simulink model "BasicFF"  (R2016a)
settings: Solver=FixedStepAuto  StartTime=0.0  StopTime=48*60  FixedStep=1  RelTol=1e-3
values from neighbouring files (symbols this model uses):
  Ki = -0.075*(1+Ki_uncertainty)    (= -0.075)    [DiabetesVariables.m]
  Ki0 = -0.075    [Qdesign.m]
  Km = 4    [DiabetesVariables.m]
  Tdi = 25    [DiabetesVariables.m]
  Tdm = 15    [DiabetesVariables.m]
  Ti = 140    [DiabetesVariables.m]
  Tm = 50    [DiabetesVariables.m]
settings Model: Creator=benma  LastModifiedBy=benma

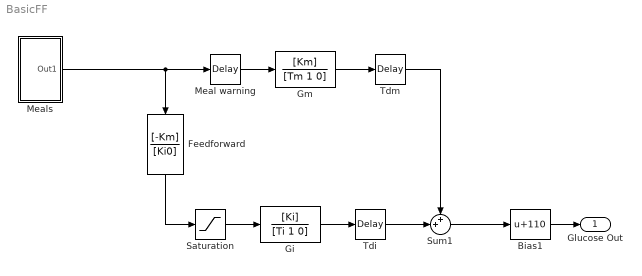
== system BasicFF ==
  Bias1 : Bias  Bias=110
  Feedforward : TransferFcn  Numerator=[-Km]  Denominator=[Ki0]
  Gi : TransferFcn  Numerator=[Ki]  Denominator=[Ti 1 0]
  Gm : TransferFcn  Numerator=[Km]  Denominator=[Tm 1 0]
  Meal warning : TransportDelay  DelayTime=10
  Meals : Subsystem
  Saturation : Saturate  UpperLimit=166  LowerLimit=0
  Sum1 : Sum  Inputs=++|
  Tdi : TransportDelay  DelayTime=Tdi
  Tdm : TransportDelay  DelayTime=Tdm
  Glucose Out : Outport
  wires:
  Gi/1 -> Tdi/1
  Tdi/1 -> Sum1/2
  Gm/1 -> Tdm/1
  Sum1/1 -> Bias1/1
  Tdm/1 -> Sum1/1
  Bias1/1 -> Glucose Out/1
  Saturation/1 -> Gi/1
  Feedforward/1 -> Saturation/1
  Meals/1(Out1) -> Meal warning/1, Feedforward/1
  Meal warning/1 -> Gm/1

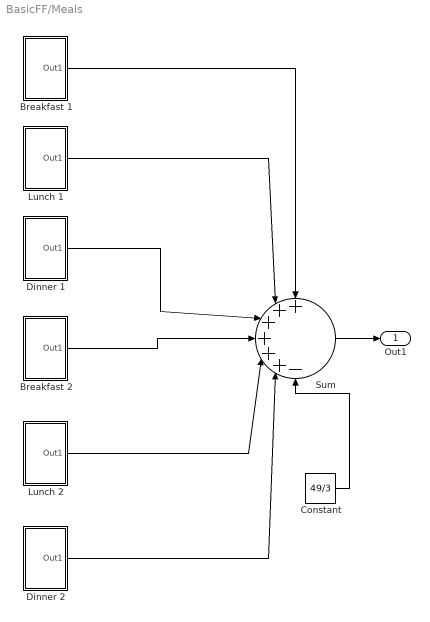
== system BasicFF/Meals ==
  Breakfast 1 : Subsystem
  Breakfast 2 : Subsystem
  Constant : Constant  Value=49/3
  Dinner 1 : Subsystem
  Dinner 2 : Subsystem
  Lunch 1 : Subsystem
  Lunch 2 : Subsystem
  Sum : Sum  Inputs=++++++-
  Out1 : Outport
  wires:
  Breakfast 1/1(Out1) -> Sum/1
  Lunch 1/1(Out1) -> Sum/2
  Dinner 1/1(Out1) -> Sum/3
  Breakfast 2/1(Out1) -> Sum/4
  Lunch 2/1(Out1) -> Sum/5
  Dinner 2/1(Out1) -> Sum/6
  Sum/1 -> Out1/1
  Constant/1 -> Sum/7

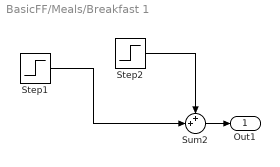
== system BasicFF/Meals/Breakfast 1 ==
  Step1 : Step  Time=60  After=25/10  SampleTime=0
  Step2 : Step  Time=70  Before=25/10  After=0  SampleTime=0
  Sum2 : Sum  Inputs=++|
  Out1 : Outport
  wires:
  Step2/1 -> Sum2/1
  Sum2/1 -> Out1/1
  Step1/1 -> Sum2/2

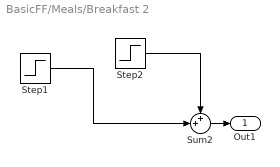
== system BasicFF/Meals/Breakfast 2 ==
  Step1 : Step  Time=25*60  After=25/10  SampleTime=0
  Step2 : Step  Time=25*60+10  Before=25/10  After=0  SampleTime=0
  Sum2 : Sum  Inputs=++|
  Out1 : Outport
  wires:
  Step2/1 -> Sum2/1
  Sum2/1 -> Out1/1
  Step1/1 -> Sum2/2

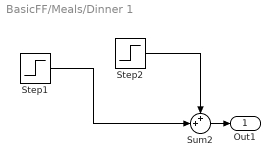
== system BasicFF/Meals/Dinner 1 ==
  Step1 : Step  Time=13*60  After=60/20  SampleTime=0
  Step2 : Step  Time=13*60+20  Before=60/20  After=0  SampleTime=0
  Sum2 : Sum  Inputs=++|
  Out1 : Outport
  wires:
  Step2/1 -> Sum2/1
  Sum2/1 -> Out1/1
  Step1/1 -> Sum2/2

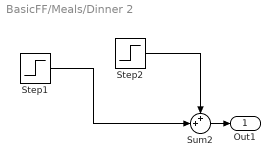
== system BasicFF/Meals/Dinner 2 ==
  Step1 : Step  Time=37*60  After=60/20  SampleTime=0
  Step2 : Step  Time=37*60+20  Before=60/20  After=0  SampleTime=0
  Sum2 : Sum  Inputs=++|
  Out1 : Outport
  wires:
  Step2/1 -> Sum2/1
  Sum2/1 -> Out1/1
  Step1/1 -> Sum2/2

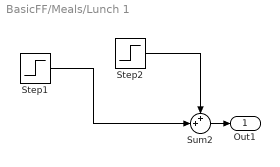
== system BasicFF/Meals/Lunch 1 ==
  Step1 : Step  Time=7*60  After=40/15  SampleTime=0
  Step2 : Step  Time=7*60+15  Before=40/15  After=0  SampleTime=0
  Sum2 : Sum  Inputs=++|
  Out1 : Outport
  wires:
  Step2/1 -> Sum2/1
  Sum2/1 -> Out1/1
  Step1/1 -> Sum2/2

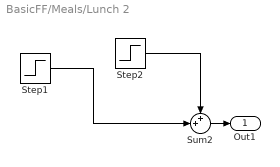
== system BasicFF/Meals/Lunch 2 ==
  Step1 : Step  Time=31*60  After=40/15  SampleTime=0
  Step2 : Step  Time=31*60+15  Before=40/15  After=0  SampleTime=0
  Sum2 : Sum  Inputs=++|
  Out1 : Outport
  wires:
  Step2/1 -> Sum2/1
  Sum2/1 -> Out1/1
  Step1/1 -> Sum2/2
